simulink model "IMC"  (R2025a)
settings: Solver=FixedStepAuto  StartTime=0.0  StopTime=0.1  FixedStep=0.00001  RelTol=1e-3
InitFcn:
  | % 单位H，实际物理模型的电机"对应轴的电感"
  | Ls = 5.19338e-5;
  | % 单位Ω，实际物理模型的电机"相电阻"
  | Rs = 0.1906689107;
  | 
  | % 单位H，预测的电机“对应轴的电感”
  | Ls_pre = 5.29338e-5;
  | % 单位Ω，预测的电机“相电阻”
  | Rs_pre = 0.2306689107;
  | 
  | % 单位rad/s，一阶低通滤波的截止频率
  | wc = 2000;
  | 
  | % 单位s秒，控制周期的大小
  | T = 0.00005;
settings Model: Creator=星必尘Sguan  LastModifiedBy=星必尘Sguan
settings SFSimCC: SimCustomHeaderCode="#include \"Sguan_InternalModel.h\""  SimCustomInitializer=SguanIMC_Init();  SimUserSources=Sguan_InternalModel.c

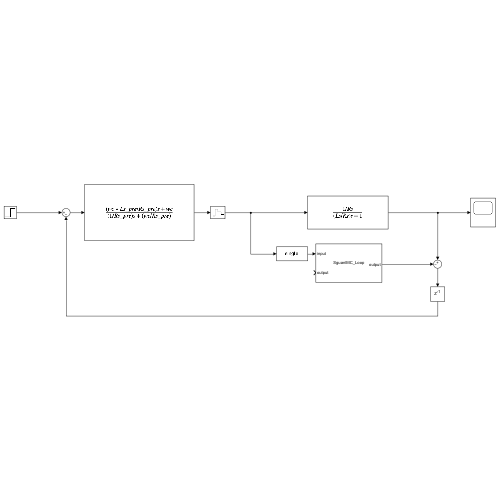
[thumbnail: Simulink's stored preview of the top-level diagram]
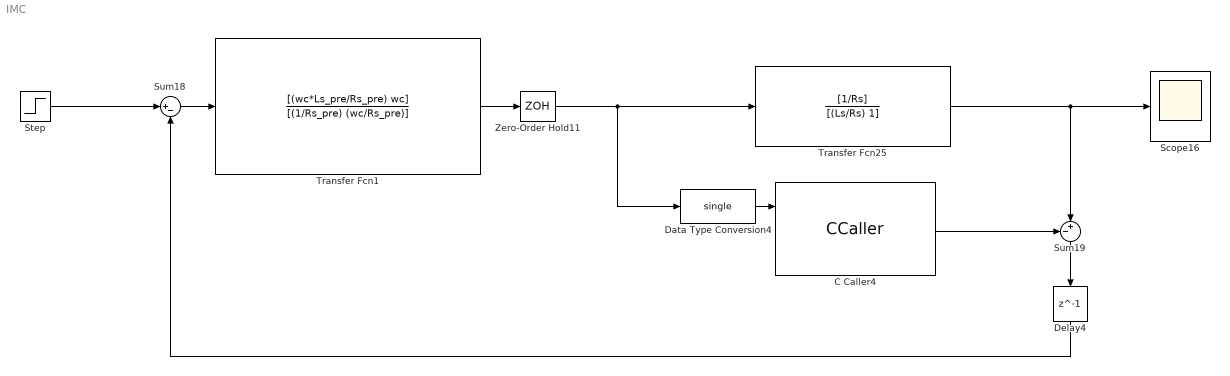
== system IMC ==
  C Caller4 : CCaller  FunctionName=SguanIMC_Loop  PortSpecificationStruct="%)30     .    X ,   8    (     @         %    \"     (    !     0         %  0 \"0    $    _    07)G3F%M90  4&]R=$YA;64 4V-O<&4     26YD97@     5'EP90      4VEZ90      27-';&]B86P   X    X    !@    @    $          4    (     0    4    !         !     %    :6YP=70    .    .     8    (    !          %    \"     $    %     0         0    !0   &EN<'5T    #@   #@    &    \"     0         !0    @    !    !0    $         $     4   !);G!U=     X    X    !@    @    &          4    (     0    $    !          D    (               .    .     8    (    !          %    \"     $    &     0         0    !@   '-I;F=L90  #@   #     &    \"     0         !0    @    !     0    $         $  ! #$    .    ,     8    (    \"0(        %    \"     $    !     0         \"  $       X    X    !@    @    $          4    (     0    8    !         !     &    ;W5T<'5T   .    .     8    (    !          %    \"     $    &     0         0    !@   &]U='!U=   #@   $     &    \"     0         !0    @    !    \"P    $         $     L   !);G!U=$]U='!U=       #@   #@    &    \"     8         !0    @    !     0    $         \"0    @           #P/PX    X    !@    @    $          4    (     0    8    !         !     &    <VEN9VQE   .    ,     8    (    !          %    \"     $    \"     0         0  ( +3$   X    P    !@    @    ) @        4    (     0    $    !          (  0"
  Data Type Conversion4 : DataTypeConversion  OutDataTypeStr=single  SaturateOnIntegerOverflow=off  RndMeth=Floor
  Delay4 : Delay  DelayLength=1
  Scope16 : Scope
      settings: ActiveDisplayYMinimum=-1.25037022221585  ActiveDisplayYMaximum=11.253331999942651  DataLoggingVariableName=ScopeData17
  Step : Step  Time=0.03  After=10  SampleTime=0
  Sum18 : Sum  Inputs=|+-
  Sum19 : Sum  Inputs=-+|
  Transfer Fcn1 : TransferFcn  Numerator=[(wc*Ls_pre/Rs_pre) wc]  Denominator=[(1/Rs_pre) (wc/Rs_pre)]
  Transfer Fcn25 : TransferFcn  Numerator=[1/Rs]  Denominator=[(Ls/Rs) 1]
  Zero-Order Hold11 : ZeroOrderHold  SampleTime=T
  wires:
  Sum18/1 -> Transfer Fcn1/1
  Sum19/1 -> Delay4/1
  Transfer Fcn25/1 -> Sum19/2, Scope16/1
  C Caller4/1 -> Sum19/1
  Step/1 -> Sum18/1
  Data Type Conversion4/1 -> C Caller4/1
  Delay4/1 -> Sum18/2
  Transfer Fcn1/1 -> Zero-Order Hold11/1
  Zero-Order Hold11/1 -> Transfer Fcn25/1, Data Type Conversion4/1
